simulink model "Read_analog_Input"  (R2018a)
settings: Solver=VariableStepAuto  StartTime=0.0  StopTime=10.0  RelTol=1e-3
libraries: arduinolib x2
settings Model: Creator=thanhdo  LastModifiedBy=thanhdo

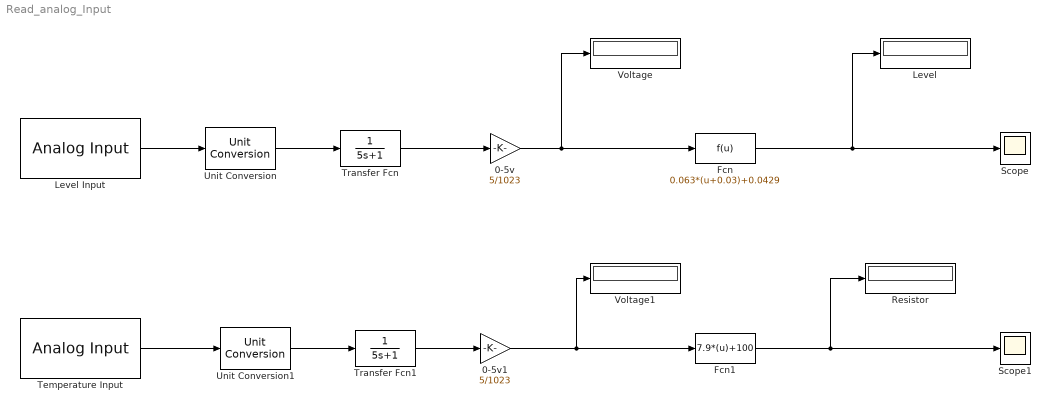
== system Read_analog_Input ==
  0-5v : Gain  Gain=5/1023
  0-5v1 : Gain  Gain=5/1023
  Fcn : Fcn  Expr=0.063*(u+0.03)+0.0429
  Fcn1 : Fcn  Expr=7.9*(u)+100
  Level : Display
  Level Input : arduinolib/Analog Input  pinNumber=4  ReadResultsOnly=off  ConversionTriggerSource=Software  ExternalTriggerType=uint32(0)  OutputDataType=uint16  EnableConversionCompleteNotify=off  EnableOuputStatus=off  SampleTime=1  blockPlatform=arduino
  Resistor : Display
  Scope : Scope
  Scope1 : Scope
  Temperature Input : arduinolib/Analog Input  pinNumber=5  ReadResultsOnly=off  ConversionTriggerSource=Software  ExternalTriggerType=uint32(0)  OutputDataType=uint16  EnableConversionCompleteNotify=off  EnableOuputStatus=off  SampleTime=1  blockPlatform=arduino
  Transfer Fcn : TransferFcn  Denominator=[5 1]
  Transfer Fcn1 : TransferFcn  Denominator=[5 1]
  Unit Conversion : UnitConversion
  Unit Conversion1 : UnitConversion
  Voltage : Display
  Voltage1 : Display
  wires:
  Level Input/1 -> Unit Conversion/1
  Unit Conversion/1 -> Transfer Fcn/1
  Transfer Fcn/1 -> 0-5v/1
  0-5v/1 -> Voltage/1, Fcn/1
  Fcn/1 -> Level/1, Scope/1
  Temperature Input/1 -> Unit Conversion1/1
  Unit Conversion1/1 -> Transfer Fcn1/1
  Transfer Fcn1/1 -> 0-5v1/1
  0-5v1/1 -> Voltage1/1, Fcn1/1
  Fcn1/1 -> Resistor/1, Scope1/1
